simulink model "rrmc_cl_01"  (R2014a)
settings: Solver=ode1  StartTime=0.0  StopTime=stop_time  FixedStep=step_time  MaxStep=0.01  RelTol=1e-3
values from neighbouring files (symbols this model uses):
  deltaTCP = [-0.08 0.2 0.03]    [rrmc_cl_pre_post_01.m]    (also in rrmc_cl_pre_post_01_CopiaProf.m = [-.3 .1 .2])
  Kp = 100    [rrmc_cl_pre_post_01.m]    (also in rrmc_cl_pre_post_01_CopiaProf.m)
  qvet_ini = [-0.0000    1.4526   -2.6861    0.0000    1.2335   -0.0000]    [rrmc_cl_pre_post_01.m]    (also in rrmc_cl_pre_post_01_CopiaProf.m = deg2rad([0 45 -30 -10 -90 -30]); rrmc_ol_pre_post_01.m = [0 0 0 0 30 0]'*pi/180)
  stop_time = 2    [rrmc_cl_pre_post_01.m]    (also in rrmc_cl_pre_post_01_CopiaProf.m = 5; rrmc_ol_pre_post_01.m = 1)
  TCP_ini = rob6R.fkine(qvet_ini)    [rrmc_cl_pre_post_01.m]    (also in rrmc_cl_pre_post_01_CopiaProf.m)
undefined symbols (not defined in the file or in its folder): transl
libraries: roblocks x4
settings Model: Creator=d029694  LastModifiedBy=Guglielmo
settings DataIOCC: LimitDataPoints=off
settings OptimizationCC: SimCompilerOptimization=off
settings DebuggingCC: MergeDetectMultiDrivingBlocksExec=error  FrameProcessingCompatibilityMsg=error
settings RTWCC: RTWCompilerOptimization=off

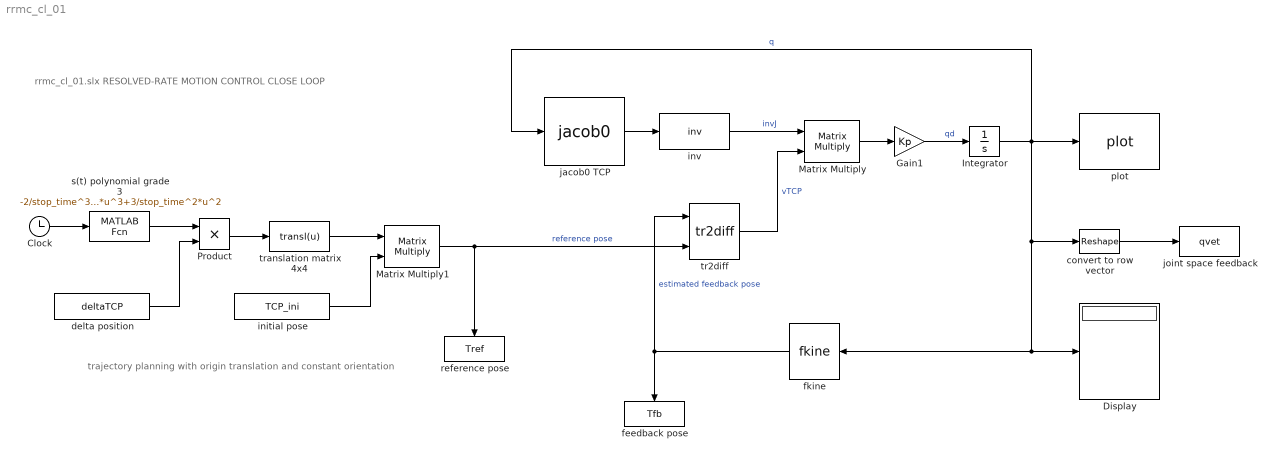
== system rrmc_cl_01 ==
  note: trajectory planning with
      | origin translation and constant orientation
  note: rrmc_cl_01.slx
      |
      | RESOLVED-RATE MOTION CONTROL
      | CLOSE LOOP
  Clock : Clock
  Display : Display
  Gain1 : Gain  Gain=Kp
  Integrator : Integrator  InitialCondition=qvet_ini
  Matrix Multiply : Product  Multiplication=Matrix(*)
  Matrix Multiply1 : Product  Multiplication=Matrix(*)
  Product : Product
  convert to row vector : Reshape  OutputDimensions=6
  delta position : Constant  Value=deltaTCP  VectorParams1D=off
  feedback pose : ToWorkspace  VariableName=Tfb  SampleTime=-1
  fkine : roblocks/Kinematics/fkine  robot=rob6R
  initial pose : Constant  Value=TCP_ini  VectorParams1D=off
  inv : MATLABFcn  MATLABFcn=inv  Output1D=off
  "jacob0 TCP " : roblocks/Kinematics/jacob0   robot=rob6R
  joint space feedback : ToWorkspace  VariableName=qvet  SampleTime=-1
  plot : roblocks/Robot Graphics/plot  robot=rob6R  fps=25  holdplot=on
  reference pose : ToWorkspace  VariableName=Tref  SampleTime=-1
  s(t) polynomial grade 3 : MATLABFcn  MATLABFcn=-2/stop_time^3*u^3+3/stop_time^2*u^2  OutputDimensions=1
  tr2diff : roblocks/Kinematics/tr2diff  robot=rob6R
  translation matrix 4x4 : MATLABFcn  MATLABFcn=transl(u)  Output1D=off
  wires:
  Integrator/1 -> fkine/1, Display/1, convert to row vector/1, "jacob0 TCP "/1, plot/1  "q"
  Matrix Multiply/1 -> Gain1/1
  "jacob0 TCP "/1 -> inv/1
  inv/1 -> Matrix Multiply/1  "invJ"
  convert to row vector/1 -> joint space feedback/1
  tr2diff/1 -> Matrix Multiply/2  "vTCP"
  fkine/1 -> feedback pose/1, tr2diff/1  "estimated feedback pose"
  Clock/1 -> s(t) polynomial grade 3/1
  initial pose/1 -> Matrix Multiply1/2
  s(t) polynomial grade 3/1 -> Product/1
  delta position/1 -> Product/2
  Product/1 -> translation matrix 4x4/1
  translation matrix 4x4/1 -> Matrix Multiply1/1
  Matrix Multiply1/1 -> tr2diff/2, reference pose/1  "reference pose"
  Gain1/1 -> Integrator/1  "qd"
